simulink library "hapsrav_library"  (R2017a)
settings: Solver=VariableStepAuto  StartTime=0.0  StopTime=10.0  RelTol=1e-3
values from neighbouring files (symbols this model uses):
  absorb_h = 0:100:40000    [EnergySim.m]
  Adisk = pi * v.R_prop^2    [EnergySim.m]
  alpha_h = absorb_h    [EnergySim.m]
  aoa_data = zeros(n_cl, n)    [EnergySim.m]
  cl_bp = linspace(min_cl, max_cl,n_cl)    [EnergySim.m]
  D = [1       -.0065      288.15          0                   101325 ... (first row only)    [EnergySim.m]    (also in msn_params.m = sqrt((from_x - to_x)^2 + (from_y - to_y)^2); solar_vector.m = time.day + ut_time)
  d2r = pi / 180    (= 0.0174532925199)    [EnergySim.m]    (also in example1.m; example2.m; example3.m; example4.m)
  d_init = sqrt(dx*dx + dy*dy)    [EnergySim.m]    (also in msn_init.m)
  dchi0 = atan2(sin(dchi0), cos(dchi0))    [EnergySim.m]    (also in msn_init.m)
  dT = 0.5    [EnergySim.m]
  dT_fixed = 0.5    [EnergySim.m]
  dT_trig = 30    [EnergySim.m]
  earth_rho = 6378137.0    (= 6378137)    [EnergySim.m]
  fp = solarFP(p.orbit_rho, p.min_axis, p.orbit_dir, ic.x_ctr, ic.y_ctr, sun_az_0)    [EnergySim.m]    (also in load_fp.m = gid_tc(msn_idx).fp; solarFP.m = [1	6	2	nul eul 0	0	0	0	1	0)
  fp_coords = [x_entry y_entry]    [msn_params.m]
  fp_courses = [chi_adj nxt_chi dchi]    [msn_params.m]
  g = 9.80665    [EnergySim.m]
  Gsolar = 1367    [EnergySim.m]
  k = k+1    (= 5)    [EnergySim.m]
  K = D(:,2)    [EnergySim.m]
  lat_init = ic.lat_init_deg * obj.d2r    [EnergySim.m]
  M = time.month    [solar_vector.m]
  max_cl = max(cl_data(:))    [EnergySim.m]
  min_cl = min(cl_data(:))    [EnergySim.m]
  ND2 = load(fullfile(pwd,'nd2_data.mat'))    [EnergySim.m]    (also in nd2_data.mat = [0.0999999999999 0.200000000001 0.3 0.4 0.499999999998 0.700)
  next_init = fp(init_wp, 3)    [EnergySim.m]    (also in msn_init.m)
  pE_init = ic.pE_init    [EnergySim.m]
  pN_init = ic.pN_init    [EnergySim.m]
  r2d = 180 / pi    (= 57.2957795131)    [EnergySim.m]    (also in example1.m; example2.m; example3.m; example4.m)
  rho_SL = 1.225    [EnergySim.m]
  S = 110.4    [EnergySim.m]
  thr_lo_lim = 0.0    (= 0)    [EnergySim.m]
  time_init = struct('year', time.year, 'month', time.month,                  'day', time.day, 'hour', time.hour, 'min', time.min,                  'UTC', time.UTC)    [EnergySim.m]
  to_init = fp(init_wp, 1)    [EnergySim.m]    (also in msn_init.m)
  vgnd_init = sqrt(Vg)    [EnergySim.m]
  vtas_init = veas_init * sqrt(rho_sl/rho_alt)    [EnergySim.m]
  w_alt = 2.0 * w_alt    [EnergySim.m]
  w_xtrack = 2.0 * w_xtrack    [EnergySim.m]
undefined symbols (not defined in the file or in its folder): alpha, alpha_bp, alpha_circ, alt0_rate_init, alt_bp, alt_cmd_mode, alt_init, alt_lim_h, alt_lim_l, alt_rt_lim_periodic, cd_data, charge_eff, chi0_rate_init, chi_cmd_mode, chi_inf, chi_init, cl_data, discharge_eff, DiscIntNeverNeededParam, E_batt_max, E_init, Earth, enableFuzzyLogic, entry_init, epsln, epsln_circ, exit_init, f8_azimuth_offset, fig_eight_time, fp0, fp_coords0, fp_courses0, gamma_lim, hold_time, k_c, K_circ, lat_init_deg, lon_init_deg, max_alpha_bp, max_alt_bp, min_alpha_bp, min_alt_bp, min_axis, motor_eff, mppt_eff, num_motors, orb_dir_init, orb_len_init, orbit_dir, orbit_rho, P_acc, panel_eff, panel_vecs, phi_0, phi_lim, phi_lim_alt, phi_lim_alt_max, phi_lim_alt_min, phi_rt_lim, prop_eff_scale ... (+39)
libraries: simulink x59, hapsrav_library x9, fuzblock x3, atmospheric_library x1, aerolibtransform2 x1
(part 1 of 6)
settings Model: Creator=benthomsen  LastModifiedBy=marriott

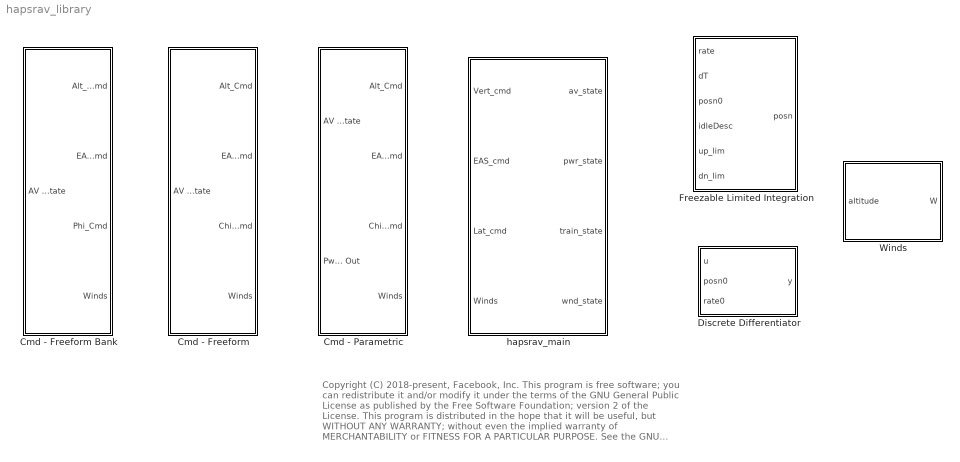
== system hapsrav_library ==
  note: Copyright (C) 2018-present, Facebook, Inc.
      |
      | This program is free software; you can redistribute it and/or modify
      | it under the terms of the GNU General Public License as published by
      | the Free Software Foundation; version 2 of the License.
      |
      | This program is distributed in the hope that it will be useful,
      | but WITHOUT ANY WARRANTY; without even the implied warranty of
      | MERCHANTABILITY or FITNESS FOR A PARTICULAR PURPOSE. See the
      | GNU General Public License for more details.
      |
      | You should have received a copy of the GNU General Public License along
      | with this program; if not, write to the Free Software Foundation, Inc.,
      | 51 Franklin Street, Fifth Floor, Boston, MA 02110-1301 USA.
  Cmd - Freeform : Subsystem
  Cmd - Freeform Bank : Subsystem
  Cmd - Parametric : Subsystem
  Discrete Differentiator : Subsystem
  Freezable Limited Integration : Subsystem
  Winds : Subsystem
  hapsrav_main : Subsystem

== system hapsrav_library/Cmd - Freeform ==
  AV State : Inport
  Alt Cmd : Subsystem
  Chi Cmd : Subsystem
  Demux1 : Demux  Outputs=28
  EAS Cmd : Subsystem
  Terminator{,1..8,10..17,19..27} (26 alike) : Terminator
  Unit Delay : UnitDelay  InitialCondition=alt_init  SampleTime=-1
  Unit Delay1 : UnitDelay  InitialCondition=chi_init  SampleTime=-1
  Winds1 : hapsrav_library/Winds
  Alt_Cmd : Outport
  EAS_Cmd : Outport  Port=2
  Chi_Cmd : Outport  Port=3
  Winds : Outport  Port=4
  wires:
  Demux1/15 -> Terminator12/1
  [alt] -> Alt Cmd/1(alt)
  Demux1/18 -> Terminator15/1
  Demux1/22 -> Terminator19/1
  Demux1/6 -> Terminator4/1
  Demux1/23 -> Terminator20/1
  Demux1/9 -> Terminator7/1
  Demux1/3 -> Terminator1/1
  Demux1/7 -> Terminator5/1
  Demux1/12 -> Unit Delay/1
  [chi] -> Chi Cmd/1(chi)
  Demux1/13 -> Terminator10/1
  Demux1/5 -> Terminator3/1
  Demux1/2 -> Terminator/1
  Demux1/20 -> Terminator17/1
  Demux1/24 -> Terminator21/1
  Demux1/10 -> Terminator8/1
  AV State/1 -> Demux1/1
  Demux1/8 -> Terminator6/1
  Demux1/16 -> Terminator13/1
  Demux1/14 -> Terminator11/1
  Demux1/19 -> Terminator16/1
  Demux1/17 -> Terminator14/1
  Demux1/4 -> Terminator2/1
  Demux1/21 -> Unit Delay1/1
  Alt Cmd/1(alt cmd) -> Alt_Cmd/1
  EAS Cmd/1(eas_cmd) -> EAS_Cmd/1
  Chi Cmd/1(chi_cmd) -> Chi_Cmd/1
  Unit Delay/1 -> [alt]
  Unit Delay1/1 -> [chi]
  Winds1/1 -> Winds/1
  [alt] -> Winds1/1
  Demux1/28 -> Terminator25/1
  Demux1/27 -> Terminator24/1
  Demux1/26 -> Terminator23/1
  Demux1/25 -> Terminator22/1
  Demux1/11 -> Terminator26/1
  Demux1/1 -> Terminator27/1

== system hapsrav_library/Cmd - Freeform Bank ==
  AV State : Inport
  Demux1 : Demux  Outputs=28
  Terminator{,1..26} (27 alike) : Terminator
  Unit Delay : UnitDelay  InitialCondition=alt_init  SampleTime=-1
  Winds1 : hapsrav_library/Winds
  alt_rt_cmd : FromWorkspace  VariableName=alt_rt_cmd  SampleTime=0
  alt_rt_cmd1 : FromWorkspace  VariableName=phi_cmd  SampleTime=0
  eas_cmd_ : FromWorkspace  VariableName=eas_cmd  SampleTime=0
  Alt_Rt_Cmd : Outport
  EAS_Cmd : Outport  Port=2
  Phi_Cmd : Outport  Port=3
  Winds : Outport  Port=4
  wires:
  alt_rt_cmd1/1 -> Phi_Cmd/1
  eas_cmd_/1 -> EAS_Cmd/1
  alt_rt_cmd/1 -> Alt_Rt_Cmd/1
  Demux1/22 -> Terminator19/1
  Demux1/7 -> Terminator5/1
  Demux1/9 -> Terminator7/1
  Demux1/21 -> Terminator18/1
  Demux1/4 -> Terminator2/1
  Demux1/14 -> Terminator11/1
  Demux1/17 -> Terminator14/1
  Demux1/19 -> Terminator16/1
  AV State/1 -> Demux1/1
  Demux1/16 -> Terminator13/1
  Demux1/8 -> Terminator6/1
  Demux1/24 -> Terminator21/1
  Demux1/10 -> Terminator8/1
  Demux1/20 -> Terminator17/1
  Demux1/13 -> Terminator10/1
  Demux1/5 -> Terminator3/1
  Demux1/15 -> Terminator12/1
  Demux1/23 -> Terminator20/1
  Demux1/2 -> Terminator/1
  Demux1/3 -> Terminator1/1
  Demux1/18 -> Terminator15/1
  Demux1/6 -> Terminator4/1
  Demux1/11 -> Terminator22/1
  Winds1/1 -> Winds/1
  Unit Delay/1 -> Winds1/1
  Demux1/1 -> Terminator9/1
  Demux1/12 -> Unit Delay/1
  Demux1/25 -> Terminator23/1
  Demux1/26 -> Terminator24/1
  Demux1/27 -> Terminator25/1
  Demux1/28 -> Terminator26/1

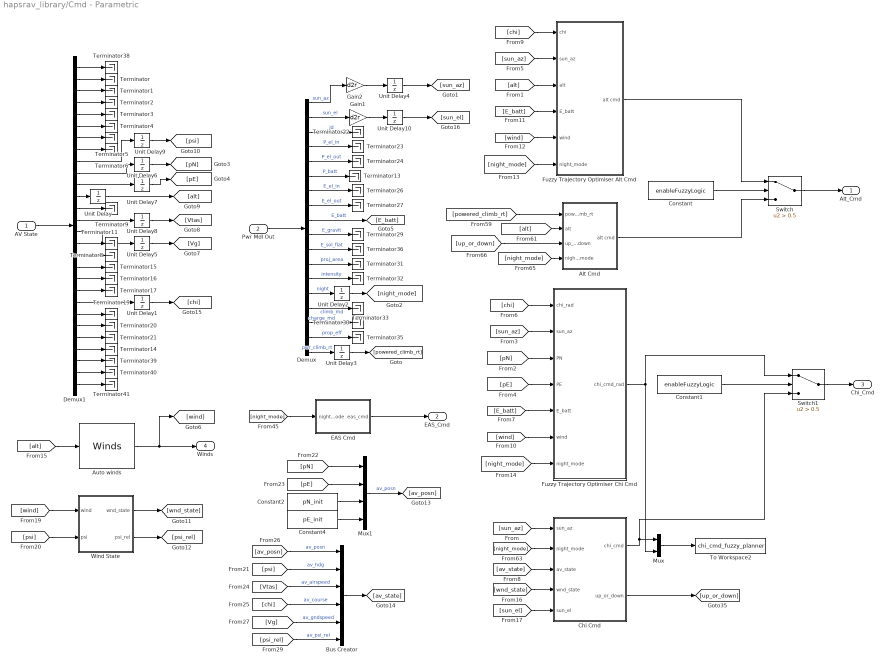
== system hapsrav_library/Cmd - Parametric ==
  AV State : Inport
  Pwr Mdl Out : Inport  Port=2
  Alt Cmd : Subsystem
  Auto winds : hapsrav_library/Winds
  Bus Creator : BusCreator  Inputs='av_posn','av_hdg','av_airspeed','av_course','av_gndspeed','av_psi_rel'
  Chi Cmd : Subsystem
  Constant : Constant  Value=enableFuzzyLogic
  Constant1 : Constant  Value=enableFuzzyLogic
  Constant2 : Constant  Value=pN_init
  Constant4 : Constant  Value=pE_init
  Demux : Demux  Outputs=18
  Demux1 : Demux  Outputs=28
  EAS Cmd : Subsystem
  Fuzzy Trajectory Optimiser Alt Cmd : Subsystem
  Fuzzy Trajectory Optimiser Chi Cmd : Subsystem
  Gain1 : Gain  Gain=d2r
  Gain2 : Gain  Gain=d2r
  Mux : Mux  Inputs=2
  Mux1 : Mux
  Switch : Switch  Criteria=u2 > Threshold  Threshold=0.5
  Switch1 : Switch  Criteria=u2 > Threshold  Threshold=0.5
  Terminator{,1..6,8..9,11,13..17,19..24,26..27,29..33,35..36,38..41} (34 alike) : Terminator
  To Workspace2 : ToWorkspace  VariableName=chi_cmd_fuzzy_planner  SampleTime=-1
  Unit Delay : UnitDelay  InitialCondition=alt_init  SampleTime=-1
  Unit Delay1 : UnitDelay  InitialCondition=chi_init  SampleTime=-1
  Unit Delay10 : UnitDelay  InitialCondition=sun_el_0  SampleTime=-1
  Unit Delay2 : UnitDelay  SampleTime=-1
  Unit Delay3 : UnitDelay  SampleTime=-1
  Unit Delay4 : UnitDelay  InitialCondition=sun_az_0  SampleTime=-1
  Unit Delay5 : UnitDelay  InitialCondition=vgnd_init  SampleTime=-1
  Unit Delay6 : UnitDelay  InitialCondition=pN_init  SampleTime=-1
  Unit Delay7 : UnitDelay  InitialCondition=pE_init  SampleTime=-1
  Unit Delay8 : UnitDelay  InitialCondition=vtas_init  SampleTime=-1
  Unit Delay9 : UnitDelay  InitialCondition=psi_0  SampleTime=-1
  Wind State : Subsystem
  Alt_Cmd : Outport
  EAS_Cmd : Outport  Port=2
  Chi_Cmd : Outport  Port=3
  Winds : Outport  Port=4
  wires:
  Gain1/1 -> Unit Delay10/1
  Demux/2 -> Gain1/1  "sun_el"
  Gain2/1 -> Unit Delay4/1
  Demux/1 -> Gain2/1  "sun_az"
  [sun_el] -> Chi Cmd/5(sun_el)
  Unit Delay10/1 -> [sun_el]
  [wnd_state] -> Chi Cmd/4(wnd_state)
  [av_state] -> Chi Cmd/3(av_state)
  [psi_rel] -> Bus Creator/6  "av_psi_rel"
  [av_posn] -> Bus Creator/1  "av_posn"
  [Vg] -> Bus Creator/5  "av_gndspeed"
  [chi] -> Bus Creator/4  "av_course"
  Bus Creator/1 -> [av_state]
  [psi] -> Bus Creator/2  "av_hdg"
  [Vtas] -> Bus Creator/3  "av_airspeed"
  [pN] -> Mux1/1
  [pE] -> Mux1/2
  Mux1/1 -> [av_posn]  "av_posn"
  Constant4/1 -> Mux1/4
  Constant2/1 -> Mux1/3
  Wind State/2(psi_rel) -> [psi_rel]
  [psi] -> Wind State/2(psi)
  Wind State/1(wnd_state) -> [wnd_state]
  [wind] -> Wind State/1(wind)
  Unit Delay9/1 -> [psi]
  Unit Delay8/1 -> [Vtas]
  Demux1/18 -> Terminator15/1
  AV State/1 -> Demux1/1
  Demux1/9 -> Unit Delay9/1
  [night_mode] -> Alt Cmd/4(night_mode)
  [up_or_down] -> Alt Cmd/3(up_or_down)
  Demux1/23 -> Terminator20/1
  [sun_az] -> Chi Cmd/1(sun_az)
  Demux1/17 -> Terminator8/1
  [night_mode] -> EAS Cmd/1(night_mode)
  Demux1/20 -> Terminator17/1
  Demux1/19 -> Terminator16/1
  Chi Cmd/2(up_or_down) -> [up_or_down]
  [powered_climb_rt] -> Alt Cmd/1(powered_climb_rt)
  Demux1/22 -> Terminator19/1
  [alt] -> Alt Cmd/2(alt)
  Demux1/4 -> Terminator2/1
  Demux1/7 -> Terminator5/1
  Demux1/5 -> Terminator3/1
  Demux1/8 -> Terminator6/1
  Demux1/10 -> Unit Delay6/1
  Demux1/2 -> Terminator/1
  Demux1/24 -> Terminator21/1
  Demux1/3 -> Terminator1/1
  Demux1/6 -> Terminator4/1
  [night_mode] -> Chi Cmd/2(night_mode)
  EAS Cmd/1(eas_cmd) -> EAS_Cmd/1
  Auto winds/1 -> [wind], Winds/1
  Unit Delay/1 -> [alt]
  Unit Delay1/1 -> [chi]
  Demux/11 -> Terminator36/1  "E_sol_flat"
  Demux/17 -> Terminator35/1  "prop_eff"
  Demux/14 -> Unit Delay2/1  "night"
  Demux/16 -> Terminator30/1  "charge_md"
  Demux/3 -> Terminator22/1  "jd"
  Pwr Mdl Out/1 -> Demux/1
  Demux/12 -> Terminator31/1  "proj_area"
  Demux/4 -> Terminator23/1  "P_el_in"
  Demux/5 -> Terminator24/1  "P_el_out"
  Demux/18 -> Unit Delay3/1  "pwr_climb_rt"
  Demux/13 -> Terminator32/1  "intensity"
  Demux/7 -> Terminator26/1  "E_el_in"
  Demux/15 -> Terminator33/1  "climb_md"
  Demux/8 -> Terminator27/1  "E_el_out"
  Demux/10 -> Terminator29/1  "E_gravit"
  Demux/9 -> [E_batt]  "E_batt"
  Demux/6 -> Terminator13/1  "P_batt"
  Unit Delay2/1 -> [night_mode]
  Unit Delay3/1 -> [powered_climb_rt]
  Unit Delay4/1 -> [sun_az]
  [chi] -> Fuzzy Trajectory Optimiser Alt Cmd/1(chi)
  [sun_az] -> Fuzzy Trajectory Optimiser Alt Cmd/2(sun_az)
  [alt] -> Fuzzy Trajectory Optimiser Alt Cmd/3(alt)
  Demux1/16 -> Terminator11/1
  Demux1/15 -> Unit Delay5/1
  Demux1/13 -> Terminator9/1
  Demux1/14 -> Unit Delay8/1
  [sun_az] -> Fuzzy Trajectory Optimiser Chi Cmd/2(sun_az)
  Mux/1 -> To Workspace2/1
  Constant/1 -> Switch/2
  Switch/1 -> Alt_Cmd/1
  Fuzzy Trajectory Optimiser Alt Cmd/1(alt cmd) -> Switch/1
  Alt Cmd/1(alt cmd) -> Switch/3
  Fuzzy Trajectory Optimiser Chi Cmd/1(chi_cmd_rad) -> Switch1/1, Mux/2
  Constant1/1 -> Switch1/2
  Switch1/1 -> Chi_Cmd/1
  Chi Cmd/1(chi_cmd) -> Switch1/3, Mux/1
  Demux1/12 -> Unit Delay/1
  Demux1/1 -> Terminator38/1
  Demux1/11 -> Unit Delay7/1
  Demux1/21 -> Unit Delay1/1
  Demux1/28 -> Terminator41/1
  Demux1/27 -> Terminator40/1
  Demux1/26 -> Terminator39/1
  Demux1/25 -> Terminator14/1
  [chi] -> Fuzzy Trajectory Optimiser Chi Cmd/1(chi_rad)
  [pN] -> Fuzzy Trajectory Optimiser Chi Cmd/3(PN)
  [pE] -> Fuzzy Trajectory Optimiser Chi Cmd/4(PE)
  [wind] -> Fuzzy Trajectory Optimiser Chi Cmd/6(wind)
  [E_batt] -> Fuzzy Trajectory Optimiser Chi Cmd/5(E_batt)
  [night_mode] -> Fuzzy Trajectory Optimiser Chi Cmd/7(night_mode)
  [E_batt] -> Fuzzy Trajectory Optimiser Alt Cmd/4(E_batt)
  [wind] -> Fuzzy Trajectory Optimiser Alt Cmd/5(wind)
  [night_mode] -> Fuzzy Trajectory Optimiser Alt Cmd/6(night_mode)
  [alt] -> Auto winds/1
  Unit Delay5/1 -> [Vg]
  Unit Delay6/1 -> [pN]
  Unit Delay7/1 -> [pE]

== system hapsrav_library/Discrete Differentiator ==
  u : Inport
  posn0 : Inport  Port=2
  rate0 : Inport  Port=3
  A : Gain  Gain=sys_lpf_A
  B : Gain  Gain=sys_lpf_B
  C : Gain  Gain=sys_lpf_C
  C1 : Gain  Gain=1/dT
  D : Gain  Gain=sys_lpf_D
  Delay : Delay  DelayLength=1  InitialConditionSource=Input port
      settings: InputPortMap=u0,p4
  Delay1 : Delay  DelayLength=1  InitialConditionSource=Input port
      settings: InputPortMap=u0,p4
  Product : Product
  Sum : Sum  Inputs=|++
  Sum1 : Sum  Inputs=|++
  Sum2 : Sum  Inputs=|+-
  x0 : Constant  Value=sys_lpf_x0
  y : Outport
  wires:
  Sum2/1 -> C1/1
  Delay1/1 -> Sum2/2
  posn0/1 -> Delay1/2
  u/1 -> Delay1/1, Sum2/1
  Delay/1 -> A/1, C/1
  Sum/1 -> Delay/1
  Sum1/1 -> y/1
  A/1 -> Sum/2
  [DuDt] -> B/1, D/1
  rate0/1 -> Product/2
  B/1 -> Sum/1
  D/1 -> Sum1/2
  x0/1 -> Product/1
  Product/1 -> Delay/2
  C/1 -> Sum1/1
  C1/1 -> [DuDt]

== system hapsrav_library/Freezable Limited Integration ==
  rate : Inport
  dT : Inport  Port=2
  posn0 : Inport  Port=3
  idleDesc : Inport  Port=4
  up_lim : Inport  Port=5
  dn_lim : Inport  Port=6
  Constant : Constant  Value=0
  Delay1 : Delay  DelayLength=1  InitialConditionSource=Input port
      settings: InputPortMap=u0,p4
  Delay2 : Delay  DelayLength=1  InitialConditionSource=Input port  InitialCondition=0
      settings: InputPortMap=u0,p4
  Delay3 : Delay  DelayLength=1  InitialConditionSource=Input port
      settings: InputPortMap=u0,p4
  Limited Integration : MATLAB Function  TreatAsAtomicUnit=on
  Switch : Switch  Threshold=1
  Switch1 : Switch  Threshold=1
  posn : Outport
  wires:
  up_lim/1 -> Limited Integration/3(uplim)
  rate/1 -> Limited Integration/1(u)
  Delay1/1 -> Limited Integration/5(x0)
  Limited Integration/2(x1) -> Delay1/1
  Limited Integration/1(y0) -> Switch/3, posn/1
  dT/1 -> Limited Integration/2(T)
  idleDesc/1 -> Delay2/1
  Delay2/1 -> [idle_desc]
  [idle_desc] -> Switch/2
  [idle_desc] -> Switch1/2
  Switch/1 -> Delay3/1
  Delay3/1 -> Switch/1, [desc_lim]
  posn0/1 -> [posn0]
  [posn0] -> Delay1/2
  [posn0] -> Delay3/2
  dn_lim/1 -> Switch1/3
  [desc_lim] -> Switch1/1
  Switch1/1 -> Limited Integration/4(lolim)
  Constant/1 -> Delay2/2

== system hapsrav_library/Winds ==
  altitude : Inport
  Constant : Constant  Value=TEST_WINDS
  Constant Winds : Subsystem
  Logical Operator : Logic  Operator=NOT  AllPortsSameDT=off  OutDataTypeStr=boolean
  Merge : Merge
  Test Winds : Subsystem
  wdir_level : Constant  Value=wdir_level
  wmag_level : Constant  Value=wmag_level
  W : Outport
  wires:
  wmag_level/1 -> Test Winds/2(wmag_level)
  wdir_level/1 -> Test Winds/3(wdir_level)
  altitude/1 -> Test Winds/1(altitude)
  Merge/1 -> W/1
  Constant Winds/1(W) -> Merge/1
  Test Winds/1(W) -> Merge/2
  Constant/1 -> Test Winds/Enable, Logical Operator/1
  Logical Operator/1 -> Constant Winds/Enable

== system hapsrav_library/hapsrav_main ==
  Vert_cmd : Inport  PortDimensions=1
  EAS_cmd : Inport  Port=2  PortDimensions=1
  Lat_cmd : Inport  Port=3  PortDimensions=1
  Winds : Inport  Port=4  PortDimensions=3
  Kinematic 6DOF : Subsystem
  Outputs : Subsystem
  av_state : Outport
  pwr_state : Outport  Port=2
  train_state : Outport  Port=3
  wnd_state : Outport  Port=4
  wires:
  Kinematic 6DOF/2(pwr_state) -> Outputs/2(Pwr State)
  Winds/1 -> Kinematic 6DOF/4(Winds)
  Lat_cmd/1 -> Kinematic 6DOF/3(Lat_cmd)
  EAS_cmd/1 -> Kinematic 6DOF/2(EAS_cmd)
  Vert_cmd/1 -> Kinematic 6DOF/1(Vert_cmd)
  Kinematic 6DOF/1(av_state) -> Outputs/1(AV State)
  Outputs/1(simOut) -> av_state/1
  Outputs/2(pwrOut) -> pwr_state/1
  Outputs/3(TrainOut) -> train_state/1
  Kinematic 6DOF/3(wnd_state) -> wnd_state/1

== system hapsrav_library/Cmd - Freeform/Alt Cmd ==
  alt : Inport
  Abs : Abs
  Compare To Constant : simulink/Logic and Bit Operations/Compare To Constant  relop=>  const=50  OutDataTypeStr=boolean
  Delay1 : Delay  DelayLength=1  InitialCondition=alt_init
  Discrete-Time Integrator : DiscreteIntegrator  IntegratorMethod=Integration: Trapezoidal  ExternalReset=rising  InitialConditionSource=external  InitialConditionSetting=State (most efficient)  SampleTime=-1  ICPrevOutput=DiscIntNeverNeededParam  ICPrevScaledInput=DiscIntNeverNeededParam
  IC : InitialCondition  Value=alt_init
  Sum : Sum  Inputs=|+-
  To Workspace : ToWorkspace  VariableName=alt_cmd  SampleTime=-1
  alt_rt_cmd : FromWorkspace  VariableName=alt_rt_cmd  SampleTime=0
  alt cmd : Outport
  wires:
  Compare To Constant/1 -> Discrete-Time Integrator/2  "trigger a reset (anti-windup)"
  Sum/1 -> Abs/1
  alt_rt_cmd/1 -> Discrete-Time Integrator/1
  alt/1 -> IC/1
  Discrete-Time Integrator/1 -> Delay1/1
  Delay1/1 -> To Workspace/1, alt cmd/1, Discrete-Time Integrator/3, Sum/2
  Abs/1 -> Compare To Constant/1
  IC/1 -> Sum/1

== system hapsrav_library/Cmd - Freeform/Chi Cmd ==
  chi : Inport
  Abs : Abs
  Compare To Constant : simulink/Logic and Bit Operations/Compare To Constant  relop=>  const=2  OutDataTypeStr=boolean
  Delay1 : Delay  DelayLength=1  InitialCondition=chi_init
  Discrete-Time Integrator : DiscreteIntegrator  IntegratorMethod=Integration: Trapezoidal  ExternalReset=rising  InitialConditionSource=external  InitialConditionSetting=State (most efficient)  SampleTime=-1  ICPrevOutput=DiscIntNeverNeededParam  ICPrevScaledInput=DiscIntNeverNeededParam
  IC : InitialCondition  Value=chi_init
  Sum : Sum  Inputs=|+-
  To Workspace : ToWorkspace  VariableName=chi_cmd  SampleTime=-1
  alt_rt_cmd : FromWorkspace  VariableName=chi_rt_cmd  SampleTime=0
  chi_cmd : Outport
  wires:
  chi/1 -> IC/1
  Delay1/1 -> To Workspace/1, chi_cmd/1, Discrete-Time Integrator/3, Sum/2
  alt_rt_cmd/1 -> Discrete-Time Integrator/1
  Abs/1 -> Compare To Constant/1
  Discrete-Time Integrator/1 -> Delay1/1
  Sum/1 -> Abs/1
  Compare To Constant/1 -> Discrete-Time Integrator/2  "trigger a reset (anti-windup)"
  IC/1 -> Sum/1

== system hapsrav_library/Cmd - Freeform/EAS Cmd ==
  eas_cmd_ : FromWorkspace  VariableName=eas_cmd  SampleTime=0
  eas_cmd : Outport
  wires:
  eas_cmd_/1 -> eas_cmd/1

== system hapsrav_library/Cmd - Parametric/Alt Cmd ==
  powered_climb_rt : Inport
  alt : Inport  Port=2
  up_or_down : Inport  Port=3
  night_mode : Inport  Port=4
  Compare To Constant : simulink/Logic and Bit Operations/Compare To Constant  relop===  const=1  OutDataTypeStr=boolean
  Compare To Constant2 : simulink/Logic and Bit Operations/Compare To Constant  relop===  const=2  OutDataTypeStr=boolean
  Constant : Constant  Value=alt_cmd_mode
  Constant2 : Constant
  Merge : Merge
  Periodic Climb/Glide : Subsystem
  Power-Limited Climb : Subsystem
  Scope : Scope
  Switch : Switch  Criteria=u2 ~= 0
  To Workspace : ToWorkspace  VariableName=alt_cmd  SampleTime=-1
  alt cmd : Outport
  wires:
  Merge/1 -> Scope/1, To Workspace/1, alt cmd/1
  powered_climb_rt/1 -> Power-Limited Climb/1(climb_rt)
  Switch/1 -> Compare To Constant2/1, Compare To Constant/1
  Compare To Constant/1 -> Power-Limited Climb/Enable
  Power-Limited Climb/1(alt_cmd) -> Merge/1
  Compare To Constant2/1 -> Periodic Climb/Glide/Enable
  Periodic Climb/Glide/1(alt_cmd) -> Merge/2
  up_or_down/1 -> Periodic Climb/Glide/1(up_or_down)
  night_mode/1 -> [night_mode]
  alt/1 -> [alt]
  [night_mode] -> Switch/2
  Constant/1 -> Switch/3
  Constant2/1 -> Switch/1
  [alt] -> Power-Limited Climb/2(alt)
  [alt] -> Periodic Climb/Glide/2(alt)

== system hapsrav_library/Cmd - Parametric/Chi Cmd ==
  sun_az : Inport
  night_mode : Inport  Port=2
  av_state : Inport  Port=3
  wnd_state : Inport  Port=4
  sun_el : Inport  Port=5
  Bus Selector : BusSelector  OutputSignals=av_hdg
  Circular Vector Fields : Subsystem  TreatAsAtomicUnit=on
  Compare To Constant1 : simulink/Logic and Bit Operations/Compare To Constant  relop===  const=4  OutDataTypeStr=boolean
  Compare To Constant2 : simulink/Logic and Bit Operations/Compare To Constant  relop===  const=5  OutDataTypeStr=boolean
  Compare To Constant3 : simulink/Logic and Bit Operations/Compare To Constant  relop===  const=3  OutDataTypeStr=boolean
  Constant2 : Constant  Value=2*pi
  Constant3 : Constant  Value=chi_cmd_mode
  Delay1 : Delay  DelayLength=1  InitialCondition=chi_init
  Flight Plan : Subsystem  TreatAsAtomicUnit=on
  Math Function1 : Math  Operator=mod  SaturateOnIntegerOverflow=on
  Merge1 : Merge  Inputs=3
  Mux4 : Mux  Inputs=2
  Scope : Scope
  Subsystem : Subsystem
  To Workspace : ToWorkspace  VariableName=chi_cmd  SampleTime=-1
  To Workspace3 : ToWorkspace  VariableName=chi_cmd_param  SampleTime=-1
  chi_cmd : Outport
  up_or_down : Outport  Port=2
  tag scope: chi_cmd=global
  wires:
  [sun_el_rad] -> Flight Plan/4(sun_el)
  sun_el/1 -> [sun_el_rad]
  Bus Selector/1 -> [chi]  "<av_hdg>"
  [av_state] -> Bus Selector/1
  [sun_az_rad] -> Flight Plan/3(sun_az)
  wnd_state/1 -> Flight Plan/2(wnd_state)
  [av_state] -> Flight Plan/1(av_state)
  Flight Plan/1(chi_ref) -> Merge1/2
  [av_state] -> Circular Vector Fields/1(av_state)
  av_state/1 -> [av_state]
  [chi_cmd_mode] -> Compare To Constant2/1
  Compare To Constant2/1 -> Flight Plan/Enable
  Compare To Constant1/1 -> Circular Vector Fields/Enable
  [chi_cmd_mode] -> Compare To Constant1/1
  Compare To Constant3/1 -> Subsystem/Enable
  [chi_cmd_mode] -> Compare To Constant3/1
  Constant3/1 -> [chi_cmd_mode]
  Subsystem/1(chi_cmd) -> Merge1/3
  Circular Vector Fields/1(chi_cmd) -> Merge1/1
  Subsystem/2(up_or_down) -> up_or_down/1
  [sun_az_rad] -> Subsystem/3(sun_az_rad)
  [chi_cmd] -> Subsystem/2(chi_cmd_in)
  [night_mode] -> Subsystem/1(night_md)
  Merge1/1 -> chi_cmd/1, Delay1/1, Scope/1, To Workspace/1, Mux4/2
  [chi] -> Mux4/1
  Mux4/1 -> Math Function1/1
  Math Function1/1 -> To Workspace3/1
  Constant2/1 -> Math Function1/2
  Delay1/1 -> [chi_cmd]
  night_mode/1 -> [night_mode]
  sun_az/1 -> [sun_az_rad]

== system hapsrav_library/Cmd - Parametric/EAS Cmd ==
  night_mode : Inport
  Constant : Constant  Value=veas_init
  Constant1 : Constant  Value=veas_night_mode
  Switch : Switch  Criteria=u2 ~= 0
  eas_cmd : Outport
  wires:
  Constant/1 -> Switch/3
  Constant1/1 -> Switch/1
  night_mode/1 -> Switch/2
  Switch/1 -> eas_cmd/1

== system hapsrav_library/Cmd - Parametric/Fuzzy Trajectory Optimiser Alt Cmd ==
  note: This is the wind vector
  chi : Inport
  sun_az : Inport  Port=2
  alt : Inport  Port=3
  E_batt : Inport  Port=4
  wind : Inport  Port=5
  night_mode : Inport  Port=6
  Alt Rate Integrator : Subsystem
  Compare To Constant1 : simulink/Logic and Bit Operations/Compare To Constant  relop=<=  const=pi  OutDataTypeStr=boolean
  Constant : Constant  Value=2*pi
  Fuzzy Logic Trajectory Planner : fuzblock/Fuzzy Logic  Controller  fis='traj_planner_altrate.fis'
  IC : InitialCondition  Value=chi_init
  "If the modulud after division is larger than pi, then sunbtract the mod results from 2*pi this procedure maps the azimuth angle difference between [0,pi]" : Switch  Criteria=u2 ~= 0
  Math Function : Math  Operator=mod  SaturateOnIntegerOverflow=on
  Mux : Mux  Inputs=2
  Subtract : Sum  Inputs=|+-
  Subtract1 : Sum  Inputs=-|+
  Terminator{,1..3} (4 alike) : Terminator
  To Workspace : ToWorkspace  VariableName=alt_cmd_fuzzy_planner  SampleTime=-1
  alt cmd : Outport
  wires:
  Fuzzy Logic Trajectory Planner/1 -> Alt Rate Integrator/1(alt_rate_cmd), Mux/1
  chi/1 -> [chi_rad], IC/1
  IC/1 -> [chi]
  [chi] -> Terminator/1
  sun_az/1 -> [sun_az_rad]
  [sun_az_rad] -> Subtract/2
  Math Function/1 -> Compare To Constant1/1, "If the modulud after division is larger than pi, then sunbtract the mod results from 2*pi this procedure maps the azimuth angle difference between [0,pi]"/1, Subtract1/1  "Azimuth difference  (rad)"
  Compare To Constant1/1 -> "If the modulud after division is larger than pi, then sunbtract the mod results from 2*pi this procedure maps the azimuth angle difference between [0,pi]"/2
  Constant/1 -> Subtract1/2, Math Function/2
  Subtract/1 -> Math Function/1
  Subtract1/1 -> "If the modulud after division is larger than pi, then sunbtract the mod results from 2*pi this procedure maps the azimuth angle difference between [0,pi]"/3
  "If the modulud after division is larger than pi, then sunbtract the mod results from 2*pi this procedure maps the azimuth angle difference between [0,pi]"/1 -> Fuzzy Logic Trajectory Planner/1
  Alt Rate Integrator/1(alt_cmd) -> Mux/2, alt cmd/1
  alt/1 -> [alt]
  [alt] -> Alt Rate Integrator/2(alt)
  Mux/1 -> To Workspace/1
  [chi_rad] -> Subtract/1
  E_batt/1 -> Terminator1/1
  wind/1 -> Terminator2/1
  night_mode/1 -> Terminator3/1

== system hapsrav_library/Cmd - Parametric/Fuzzy Trajectory Optimiser Chi Cmd ==
  note: This is the wind vector
  note: check if the aircraft is closed to the station
      |  keeping circle perimeter
  note: distance from the perimeter in meter
  chi_rad : Inport
  sun_az : Inport  Port=2
  PN : Inport  Port=3
  PE : Inport  Port=4
  E_batt : Inport  Port=5
  wind : Inport  Port=6
  night_mode : Inport  Port=7
  Abs : Abs
  Compare To Constant : simulink/Logic and Bit Operations/Compare To Constant  relop=<=  const=350  OutDataTypeStr=boolean
  Compare To Constant1 : simulink/Logic and Bit Operations/Compare To Constant  relop=<=  const=pi  OutDataTypeStr=boolean
  Constant : Constant  Value=2*pi
  Constant1 : Constant  Value=2500
  Constant2 : Constant  Value=2*pi
  Constant3 : Constant  Value=2*pi
  Discrete Derivative : simulink/Discrete/Discrete Derivative  gainval=1  ICPrevScaledInput=0.0  OutMin=[]  OutMax=[]  OutDataType=fixdt(1, 16)  OutScaling=2^-10  DoSatur=off
  Fcn : Fcn  Expr=(u(1)*u(1)+u(2)*u(2))^0.5
  Fuzzy Logic Trajectory Planner : fuzblock/Fuzzy Logic  Controller  fis='traj_planner_chi_radii.fis'
  Fuzzy Logic Trajectory Planner1 : fuzblock/Fuzzy Logic  Controller  fis='traj_planner_chi_solar.fis'
  Gain : Gain  Gain=-1
  Gain2 : Gain  Gain=1/d2r
  IC : InitialCondition  Value=chi_init
  "If the modulus after division is larger than pi, then sunbtract the mod results from 2*pi this procedure maps the azimuth angle difference between [0,pi]" : Switch  Criteria=u2 ~= 0
  "If the modulus after division is larger than pi, then sunbtract the mod results from 2*pi this procedure maps the azimuth angle difference between [0,pi]1" : Switch  Criteria=u2 > Threshold
  Math Function : Math  Operator=mod  SaturateOnIntegerOverflow=on
  Math Function1 : Math  Operator=mod  SaturateOnIntegerOverflow=on
  Math Function2 : Math  Operator=mod  SaturateOnIntegerOverflow=on
  Mux1 : Mux  Inputs=2
  Mux2 : Mux  Inputs=3
  Mux3 : Mux
  Mux4 : Mux  Inputs=2
  Subsystem : Subsystem
  Subtract : Sum  Inputs=|+-
  Subtract1 : Sum  Inputs=-|+
  Subtract2 : Sum  Inputs=-+|
  Switch : Switch  Criteria=u2 > Threshold
  Terminator{,1..3} (4 alike) : Terminator
  To Workspace1 : ToWorkspace  VariableName=chirate_cmd_vector  SampleTime=-1
  To Workspace2 : ToWorkspace  VariableName=posdiff_vector  SampleTime=-1
  To Workspace3 : ToWorkspace  VariableName=chi_cmd_fuzzy  SampleTime=-1
  chi_cmd_rad : Outport
  wires:
  sun_az/1 -> [sun_az_rad]
  Compare To Constant1/1 -> "If the modulus after division is larger than pi, then sunbtract the mod results from 2*pi this procedure maps the azimuth angle difference between [0,pi]"/2
  [sun_az_rad] -> Subtract/2
  Constant/1 -> Subtract1/2, Math Function/2
  Math Function/1 -> Compare To Constant1/1, "If the modulus after division is larger than pi, then sunbtract the mod results from 2*pi this procedure maps the azimuth angle difference between [0,pi]"/1, Subtract1/1  "Azimuth difference  (rad)"
  IC/1 -> [chi_init]
  Subtract1/1 -> "If the modulus after division is larger than pi, then sunbtract the mod results from 2*pi this procedure maps the azimuth angle difference between [0,pi]"/3
  "If the modulus after division is larger than pi, then sunbtract the mod results from 2*pi this procedure maps the azimuth angle difference between [0,pi]"/1 -> Mux2/1
  Subtract2/1 -> Mux2/2, Discrete Derivative/1, Abs/1
  PN/1 -> Mux1/1
  PE/1 -> Mux1/2
  Mux1/1 -> Fcn/1
  Fcn/1 -> Subtract2/1
  Constant1/1 -> Subtract2/2
  Mux2/1 -> Fuzzy Logic Trajectory Planner/1, Fuzzy Logic Trajectory Planner1/1
  Subsystem/1(chi_cmd_rad) -> chi_cmd_rad/1, Mux4/2
  Discrete Derivative/1 -> Mux2/3, To Workspace2/1
  chi_rad/1 -> [chi_rad], IC/1
  [chi_init] -> Terminator/1
  [chi_rad] -> Subsystem/2(chi)
  Abs/1 -> Compare To Constant/1
  Compare To Constant/1 -> Switch/2
  Switch/1 -> Mux3/3, Subsystem/1(chi_rate_cmd_rps)
  Mux3/1 -> To Workspace1/1
  Constant2/1 -> Math Function1/2
  Mux4/1 -> Math Function1/1
  [chi_rad] -> Mux4/1
  Math Function1/1 -> To Workspace3/1
  [chi_rad] -> Math Function2/1
  Constant3/1 -> Math Function2/2
  Math Function2/1 -> Subtract/1
  Fuzzy Logic Trajectory Planner/1 -> Switch/1
  Gain/1 -> "If the modulus after division is larger than pi, then sunbtract the mod results from 2*pi this procedure maps the azimuth angle difference between [0,pi]1"/1
  "If the modulus after division is larger than pi, then sunbtract the mod results from 2*pi this procedure maps the azimuth angle difference between [0,pi]1"/1 -> Mux3/1
  Subtract/1 -> "If the modulus after division is larger than pi, then sunbtract the mod results from 2*pi this procedure maps the azimuth angle difference between [0,pi]1"/2, Gain2/1, Math Function/1
  Gain2/1 -> Mux3/4
  Fuzzy Logic Trajectory Planner1/1 -> "If the modulus after division is larger than pi, then sunbtract the mod results from 2*pi this procedure maps the azimuth angle difference between [0,pi]1"/3, Mux3/2, Switch/3, Gain/1
  E_batt/1 -> Terminator1/1
  wind/1 -> Terminator2/1
  night_mode/1 -> Terminator3/1

== system hapsrav_library/Cmd - Parametric/Wind State ==
  wind : Inport
  psi : Inport  Port=2
  Demux2 : Demux  Outputs=3
  Mux1 : Mux  Inputs=2
  Product : Product
  Product1 : Product
  Rel Hdg : Subsystem
  Sqrt : Sqrt  SaturateOnIntegerOverflow=on
  Sum : Sum  Inputs=|++
  Terminator7 : Terminator
  Trigonometric Function : Trigonometry  Operator=atan2
  wnd_state : Outport
  psi_rel : Outport  Port=2
  wires:
  [Wn] -> Trigonometric Function/2
  [We] -> Trigonometric Function/1
  [Wdir] -> Rel Hdg/1(wnd_dir)
  Rel Hdg/1(rel_wnd) -> psi_rel/1
  psi/1 -> Rel Hdg/2(psi)
  [Wn] -> Product/1
  [We] -> Product1/2
  wind/1 -> Demux2/1
  Mux1/1 -> wnd_state/1
  Trigonometric Function/1 -> [Wdir]
  Demux2/3 -> Terminator7/1
  Product/1 -> Sum/1
  Sqrt/1 -> [Wspd]
  [Wdir] -> Mux1/2
  Sum/1 -> Sqrt/1
  [We] -> Product1/1
  [Wspd] -> Mux1/1
  Demux2/1 -> [Wn]
  Product1/1 -> Sum/2
  [Wn] -> Product/2
  Demux2/2 -> [We]

== system hapsrav_library/Winds/Constant Winds ==
  Enable : EnablePort
  Down : Constant  Value=Wd
  East : Constant  Value=We
  Mux : Mux  Inputs=3
  North : Constant  Value=Wn
  W : Outport
  wires:
  Down/1 -> Mux/3
  Mux/1 -> W/1
  North/1 -> Mux/1
  East/1 -> Mux/2

== system hapsrav_library/Winds/Test Winds ==
  altitude : Inport
  wmag_level : Inport  Port=2
  wdir_level : Inport  Port=3
  Enable : EnablePort
  Day : Constant  Value=wind_day
  Down : Constant  Value=Wd
  If : If  IfExpression=u1 <= 0.01
  Merge : Merge
  Merge1 : Merge
  Mux : Mux  Inputs=3
  Turn winds off at runtime : Subsystem  TreatAsAtomicUnit=on
  Winds : Subsystem  TreatAsAtomicUnit=on
  W : Outport
  wires:
  Mux/1 -> W/1
  Down/1 -> Mux/3
  [winds_on] -> Winds/Action
  Day/1 -> Winds/1(day)
  wmag_level/1 -> [wmag_level]
  [winds_off] -> Turn winds off at runtime/Action
  If/1 -> [winds_off]
  If/2 -> [winds_on]
  [wmag_level] -> If/1
  altitude/1 -> Winds/4(altitude)
  [wn_0] -> Merge/1
  [wn_1] -> Merge/2
  [we_0] -> Merge1/1
  [we_1] -> Merge1/2
  Turn winds off at runtime/1(Wn) -> [wn_0]
  Turn winds off at runtime/2(We) -> [we_0]
  Winds/1(Wn) -> [wn_1]
  Winds/2(We) -> [we_1]
  Merge1/1 -> Mux/2
  Merge/1 -> Mux/1
  [wmag_level] -> Winds/2(wmag_level)
  wdir_level/1 -> Winds/3(wdir_level)

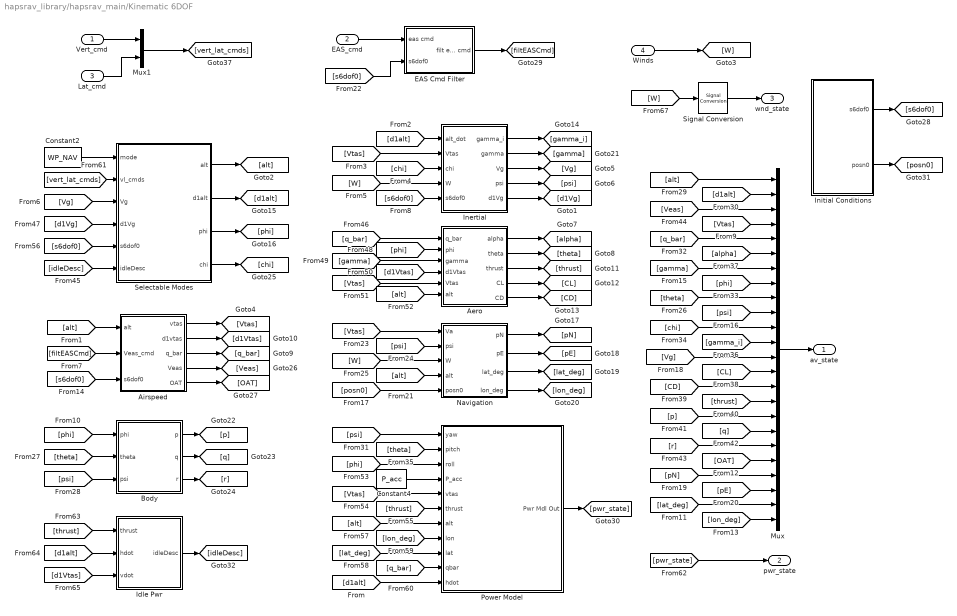
== system hapsrav_library/hapsrav_main/Kinematic 6DOF ==
  Vert_cmd : Inport
  EAS_cmd : Inport  Port=2
  Lat_cmd : Inport  Port=3
  Winds : Inport  Port=4
  Aero : Subsystem
  Airspeed : Subsystem
  Body : Subsystem
  Constant2 : Constant  Value=WP_NAV
  Constant4 : Constant  Value=P_acc
  EAS Cmd Filter : Subsystem
  Idle Pwr : Subsystem
  Inertial : Subsystem
  Initial Conditions : Subsystem
  Mux : Mux  Inputs=24
  Mux1 : Mux  Inputs=2
  Navigation : Subsystem
  Power Model : Subsystem
  Selectable Modes : Subsystem
  Signal Conversion : SignalConversion  OverrideOpt=off
  av_state : Outport
  pwr_state : Outport  Port=2
  wnd_state : Outport  Port=3
  wires:
  [s6dof0] -> Airspeed/3(s6dof0)
  [alt] -> Airspeed/1(alt)
  [filtEASCmd] -> Airspeed/2(Veas_cmd)
  Airspeed/5(OAT) -> [OAT]
  Airspeed/4(Veas) -> [Veas]
  Airspeed/3(q_bar) -> [q_bar]
  Airspeed/2(d1vtas) -> [d1Vtas]
  Airspeed/1(vtas) -> [Vtas]
  Idle Pwr/1(idleDesc) -> [idleDesc]
  [d1Vtas] -> Idle Pwr/3(vdot)
  [d1alt] -> Idle Pwr/2(hdot)
  [thrust] -> Idle Pwr/1(thrust)
  [idleDesc] -> Selectable Modes/6(idleDesc)
  Body/1(p) -> [p]
  [d1alt] -> Inertial/1(alt_dot)
  [Vtas] -> Inertial/2(Vtas)
  [chi] -> Inertial/3(chi)
  [Vtas] -> Navigation/1(Va)
  Navigation/2(pE) -> [pE]
  [phi] -> Body/1(phi)
  [theta] -> Body/2(theta)
  [psi] -> Body/3(psi)
  [W] -> Navigation/3(W)
  Inertial/1(gamma_i) -> [gamma_i]
  Inertial/4(psi) -> [psi]
  Inertial/2(gamma) -> [gamma]
  [W] -> Inertial/4(W)
  Navigation/1(pN) -> [pN]
  [psi] -> Navigation/2(psi)
  Inertial/3(Vg) -> [Vg]
  Body/2(q) -> [q]
  Body/3(r) -> [r]
  Winds/1 -> [W]
  [d1alt] -> Mux/2
  [Veas] -> Mux/3
  [Vtas] -> Mux/4
  [q_bar] -> Mux/5
  [alpha] -> Mux/6
  [gamma] -> Mux/7
  [phi] -> Mux/8
  [theta] -> Mux/9
  [psi] -> Mux/10
  [chi] -> Mux/11
  [gamma_i] -> Mux/12
  [Vg] -> Mux/13
  [CL] -> Mux/14
  [p] -> Mux/17
  [q] -> Mux/18
  [r] -> Mux/19
  Mux/1 -> av_state/1
  [alt] -> Mux/1
  [CD] -> Mux/15
  [thrust] -> Mux/16
  EAS_cmd/1 -> EAS Cmd Filter/1(eas cmd)
  EAS Cmd Filter/1(filt eas cmd) -> [filtEASCmd]
  [q_bar] -> Aero/1(q_bar)
  [phi] -> Aero/2(phi)
  [gamma] -> Aero/3(gamma)
  [d1Vtas] -> Aero/4(d1Vtas)
  [Vtas] -> Aero/5(Vtas)
  [alt] -> Aero/6(alt)
  Aero/1(alpha) -> [alpha]
  Aero/2(theta) -> [theta]
  Aero/3(thrust) -> [thrust]
  Aero/4(CL) -> [CL]
  Aero/5(CD) -> [CD]
  [alt] -> Navigation/4(alt)
  Navigation/3(lat_deg) -> [lat_deg]
  Navigation/4(lon_deg) -> [lon_deg]
  [lon_deg] -> Mux/24
  [lat_deg] -> Mux/23
  [OAT] -> Mux/20
  [pN] -> Mux/21
  [pE] -> Mux/22
  [posn0] -> Navigation/5(posn0)
  Initial Conditions/2(posn0) -> [posn0]
  Vert_cmd/1 -> Mux1/1
  Lat_cmd/1 -> Mux1/2
  Mux1/1 -> [vert_lat_cmds]
  Inertial/5(d1Vg) -> [d1Vg]
  Constant2/1 -> Selectable Modes/1(mode)
  [vert_lat_cmds] -> Selectable Modes/2(vl_cmds)
  [Vg] -> Selectable Modes/3(Vg)
  [d1Vg] -> Selectable Modes/4(d1Vg)
  [s6dof0] -> Selectable Modes/5(s6dof0)
  Selectable Modes/1(alt) -> [alt]
  Selectable Modes/2(d1alt) -> [d1alt]
  Selectable Modes/3(phi) -> [phi]
  Selectable Modes/4(chi) -> [chi]
  Initial Conditions/1(s6dof0) -> [s6dof0]
  [s6dof0] -> Inertial/5(s6dof0)
  [s6dof0] -> EAS Cmd Filter/2(s6dof0)
  [psi] -> Power Model/1(yaw)
  [d1alt] -> Power Model/11(hdot)
  [q_bar] -> Power Model/10(qbar)
  [lat_deg] -> Power Model/9(lat)
  [lon_deg] -> Power Model/8(lon)
  [alt] -> Power Model/7(alt)
  [thrust] -> Power Model/6(thrust)
  [Vtas] -> Power Model/5(vtas)
  Constant4/1 -> Power Model/4(P_acc)
  [phi] -> Power Model/3(roll)
  [theta] -> Power Model/2(pitch)
  [pwr_state] -> pwr_state/1
  [W] -> Signal Conversion/1
  Signal Conversion/1 -> wnd_state/1
  Power Model/1(Pwr Mdl Out) -> [pwr_state]

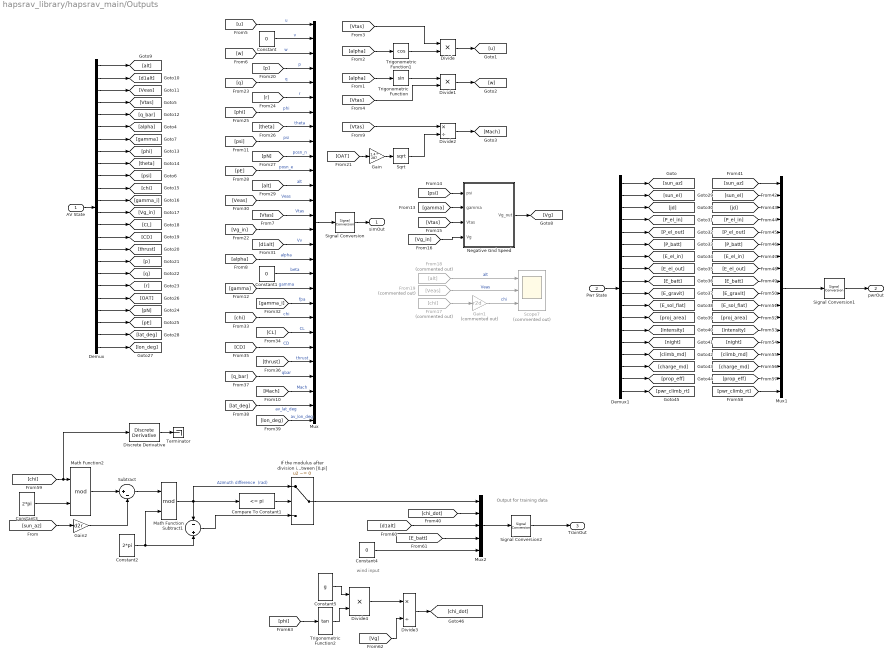
== system hapsrav_library/hapsrav_main/Outputs ==
  note: wind input
  note: Output for training data
  AV State : Inport
  Pwr State : Inport  Port=2
  Compare To Constant1 : simulink/Logic and Bit Operations/Compare To Constant  relop=<=  const=pi  OutDataTypeStr=boolean
  Constant : Constant  Value=0
  Constant1 : Constant  Value=0
  Constant2 : Constant  Value=2*pi
  Constant3 : Constant  Value=2*pi
  Constant4 : Constant  Value=0
  Constant5 : Constant  Value=g
  Demux : Demux  Outputs=24
  Demux1 : Demux  Outputs=18
  Discrete Derivative : simulink/Discrete/Discrete Derivative  gainval=1  ICPrevScaledInput=0.0  OutMin=[]  OutMax=[]  OutDataType=fixdt(1, 16)  OutScaling=2^-10  DoSatur=off
  Divide : Product  Inputs=**
  Divide1 : Product  Inputs=**
  Divide2 : Product  Inputs=*/
  Divide3 : Product  Inputs=*/
  Divide4 : Product  Inputs=**
  From17 : From  Commented=on  GotoTag=chi
  From18 : From  Commented=on  GotoTag=alt
  From19 : From  Commented=on  GotoTag=Veas
  Gain : Gain  Gain=1.4 * 287
  Gain1 : Gain  Commented=on  Gain=r2d
  Gain2 : Gain  Gain=d2r
  "If the modulus after division is larger than pi, then sunbtract the mod results from 2*pi this procedure maps the azimuth angle difference between [0,pi]" : Switch  Criteria=u2 ~= 0
  Math Function : Math  Operator=mod  SaturateOnIntegerOverflow=on
  Math Function2 : Math  Operator=mod  SaturateOnIntegerOverflow=on
  Mux : Mux  Inputs=28
  Mux1 : Mux  Inputs=18
  Mux2 : Mux  Inputs=5
  Negative Gnd Speed : Subsystem
  Scope7 : Scope  Commented=on  NumInputPorts=3
  Signal Conversion : SignalConversion  OverrideOpt=off
  Signal Conversion1 : SignalConversion  OverrideOpt=off
  Signal Conversion2 : SignalConversion  OverrideOpt=off
  Sqrt : Sqrt  SaturateOnIntegerOverflow=on
  Subtract : Sum  Inputs=|+-
  Subtract1 : Sum  Inputs=-|+
  Terminator : Terminator
  Trigonometric Function : Trigonometry
  Trigonometric Function1 : Trigonometry  Operator=cos
  Trigonometric Function2 : Trigonometry  Operator=tan
  simOut : Outport
  pwrOut : Outport  Port=2
  TrainOut : Outport  Port=3
  wires:
  [alpha] -> Trigonometric Function/1
  [alpha] -> Trigonometric Function1/1
  Trigonometric Function1/1 -> Divide/2
  [Vtas] -> Divide/1
  Trigonometric Function/1 -> Divide1/1
  [Vtas] -> Divide1/2
  Divide/1 -> [u]
  Divide1/1 -> [w]
  [u] -> Mux/1  "u"
  [w] -> Mux/3  "w"
  Constant/1 -> Mux/2  "v"
  [p] -> Mux/4  "p"
  [q] -> Mux/5  "q"
  [r] -> Mux/6  "r"
  [phi] -> Mux/7  "phi"
  [theta] -> Mux/8  "theta"
  [pN] -> Mux/10  "posn_n"
  [pE] -> Mux/11  "posn_e"
  [alt] -> Mux/12  "alt"
  [Veas] -> Mux/13  "Veas"
  [Vtas] -> Mux/14  "Vtas"
  [d1alt] -> Mux/16  "Vv"
  [alpha] -> Mux/17  "alpha"
  Constant1/1 -> Mux/18  "beta"
  [gamma_i] -> Mux/20  "fpa"
  [chi] -> Mux/21  "chi"
  [CL] -> Mux/22  "CL"
  [CD] -> Mux/23  "CD"
  [thrust] -> Mux/24  "thrust"
  [q_bar] -> Mux/25  "qbar"
  [OAT] -> Gain/1
  Gain/1 -> Sqrt/1
  [Vtas] -> Divide2/1
  Sqrt/1 -> Divide2/2
  Divide2/1 -> [Mach]
  [Mach] -> Mux/26  "Mach"
  [psi] -> Mux/9  "psi"
  [gamma] -> Mux/19  "gamma"
  [psi] -> Negative Gnd Speed/1(psi)
  [gamma] -> Negative Gnd Speed/2(gamma)
  [Vtas] -> Negative Gnd Speed/3(Vtas)
  Negative Gnd Speed/1(Vg_out) -> [Vg]
  From17/1 -> Gain1/1
  From18/1 -> Scope7/1  "alt"
  From19/1 -> Scope7/2  "Veas"
  Gain1/1 -> Scope7/3  "chi"
  AV State/1 -> Demux/1
  Demux/4 -> [Vtas]
  Demux/6 -> [alpha]
  Demux/7 -> [gamma]
  Demux/10 -> [psi]
  Demux/2 -> [d1alt]
  Demux/3 -> [Veas]
  Demux/5 -> [q_bar]
  Demux/8 -> [phi]
  Demux/9 -> [theta]
  Demux/15 -> [CD]
  Demux/16 -> [thrust]
  Demux/11 -> [chi]
  Demux/12 -> [gamma_i]
  Demux/13 -> [Vg_in]
  Demux/14 -> [CL]
  Demux/17 -> [p]
  Demux/18 -> [q]
  Demux/19 -> [r]
  Demux/20 -> [OAT]
  Demux/21 -> [pN]
  Demux/22 -> [pE]
  Demux/23 -> [lat_deg]
  Demux/24 -> [lon_deg]
  [lat_deg] -> Mux/27  "av_lat_deg"
  [lon_deg] -> Mux/28  "av_lon_deg"
  Demux/1 -> [alt]
  Mux/1 -> Signal Conversion/1
  Signal Conversion/1 -> simOut/1
  Signal Conversion1/1 -> pwrOut/1
  Gain2/1 -> Subtract/2
  Constant3/1 -> Math Function2/2
  Math Function/1 -> Compare To Constant1/1, "If the modulus after division is larger than pi, then sunbtract the mod results from 2*pi this procedure maps the azimuth angle difference between [0,pi]"/1, Subtract1/1  "Azimuth difference  (rad)"
  [chi] -> Discrete Derivative/1, Math Function2/1
  Math Function2/1 -> Subtract/1
  Subtract/1 -> Math Function/1
  Subtract1/1 -> "If the modulus after division is larger than pi, then sunbtract the mod results from 2*pi this procedure maps the azimuth angle difference between [0,pi]"/3
  Constant2/1 -> Subtract1/2, Math Function/2
  Compare To Constant1/1 -> "If the modulus after division is larger than pi, then sunbtract the mod results from 2*pi this procedure maps the azimuth angle difference between [0,pi]"/2
  Demux1/1 -> [sun_az]
  Pwr State/1 -> Demux1/1
  Demux1/2 -> [sun_el]
  Demux1/3 -> [jd]
  Demux1/4 -> [P_el_in]
  Demux1/5 -> [P_el_out]
  Demux1/6 -> [P_batt]
  Demux1/7 -> [E_el_in]
  Demux1/8 -> [E_el_out]
  Demux1/9 -> [E_batt]
  Demux1/10 -> [E_gravit]
  Demux1/11 -> [E_sol_flat]
  Demux1/12 -> [proj_area]
  Demux1/13 -> [intensity]
  Demux1/14 -> [night]
  Demux1/15 -> [climb_md]
  Demux1/16 -> [charge_md]
  Demux1/17 -> [prop_eff]
  Demux1/18 -> [pwr_climb_rt]
  [jd] -> Mux1/3
  [climb_md] -> Mux1/15
  [intensity] -> Mux1/13
  [P_el_out] -> Mux1/5
  [E_batt] -> Mux1/9
  [P_el_in] -> Mux1/4
  [proj_area] -> Mux1/12
  [sun_az] -> Mux1/1
  [P_batt] -> Mux1/6
  [E_sol_flat] -> Mux1/11
  [night] -> Mux1/14
  [E_gravit] -> Mux1/10
  [pwr_climb_rt] -> Mux1/18
  [E_el_in] -> Mux1/7
  [prop_eff] -> Mux1/17
  [sun_el] -> Mux1/2
  [E_el_out] -> Mux1/8
  [charge_md] -> Mux1/16
  Mux1/1 -> Signal Conversion1/1
  "If the modulus after division is larger than pi, then sunbtract the mod results from 2*pi this procedure maps the azimuth angle difference between [0,pi]"/1 -> Mux2/1
  [sun_az] -> Gain2/1
  Mux2/1 -> Signal Conversion2/1
  Signal Conversion2/1 -> TrainOut/1
  [chi_dot] -> Mux2/2
  [d1alt] -> Mux2/3
  [E_batt] -> Mux2/4
  Constant4/1 -> Mux2/5
  Trigonometric Function2/1 -> Divide4/2
  [phi] -> Trigonometric Function2/1
  Discrete Derivative/1 -> Terminator/1
  Constant5/1 -> Divide4/1
  Divide4/1 -> Divide3/1
  [Vg] -> Divide3/2
  Divide3/1 -> [chi_dot]
  [Vg_in] -> Mux/15
  [Vg_in] -> Negative Gnd Speed/4(Vg)

== system hapsrav_library/Cmd - Parametric/Alt Cmd/Periodic Climb//Glide ==
  up_or_down : Inport
  alt : Inport  Port=2
  Enable : EnablePort
  Abs : Abs
  Compare To Constant : simulink/Logic and Bit Operations/Compare To Constant  relop=>  const=50  OutDataTypeStr=boolean
  Delay1 : Delay  DelayLength=1  InitialCondition=alt_init
  Discrete-Time Integrator : DiscreteIntegrator  IntegratorMethod=Integration: Trapezoidal  ExternalReset=rising  InitialConditionSource=external  InitialConditionSetting=State (most efficient)  SampleTime=-1  ICPrevOutput=DiscIntNeverNeededParam  ICPrevScaledInput=DiscIntNeverNeededParam
  Gain : Gain  Gain=alt_rt_lim_periodic
  Sum : Sum  Inputs=|+-
  alt_cmd : Outport
  wires:
  Delay1/1 -> alt_cmd/1, Discrete-Time Integrator/3, Sum/2
  Compare To Constant/1 -> Discrete-Time Integrator/2  "trigger a reset (anti-windup)"
  Sum/1 -> Abs/1
  up_or_down/1 -> Gain/1
  alt/1 -> Sum/1
  Discrete-Time Integrator/1 -> Delay1/1
  Abs/1 -> Compare To Constant/1
  Gain/1 -> Discrete-Time Integrator/1

== system hapsrav_library/Cmd - Parametric/Alt Cmd/Power-Limited Climb ==
  climb_rt : Inport
  alt : Inport  Port=2
  Enable : EnablePort
  Abs : Abs
  Compare To Constant : simulink/Logic and Bit Operations/Compare To Constant  relop=>  const=50  OutDataTypeStr=boolean
  Delay1 : Delay  DelayLength=1  InitialCondition=alt_init
  Discrete-Time Integrator : DiscreteIntegrator  IntegratorMethod=Integration: Trapezoidal  ExternalReset=rising  InitialConditionSource=external  InitialConditionSetting=State (most efficient)  SampleTime=-1  ICPrevOutput=DiscIntNeverNeededParam  ICPrevScaledInput=DiscIntNeverNeededParam
  Sum : Sum  Inputs=|+-
  alt_cmd : Outport
  wires:
  Delay1/1 -> alt_cmd/1, Discrete-Time Integrator/3, Sum/2
  Compare To Constant/1 -> Discrete-Time Integrator/2  "trigger a reset (anti-windup)"
  Sum/1 -> Abs/1
  alt/1 -> Sum/1
  Discrete-Time Integrator/1 -> Delay1/1
  Abs/1 -> Compare To Constant/1
  climb_rt/1 -> Discrete-Time Integrator/1

== system hapsrav_library/Cmd - Parametric/Chi Cmd/Circular Vector Fields ==
  av_state : Inport
  Enable : EnablePort  StatesWhenEnabling=reset
  Bus Selector : BusSelector  OutputSignals=av_posn,av_course,av_gndspeed
  Constant1 : Constant  Value=x_ctr
  Constant12 : Constant  Value=k_c
  Constant2 : Constant  Value=epsln_circ
  Constant3 : Constant  Value=y_ctr
  Constant4 : Constant  Value=alpha_circ
  Constant5 : Constant  Value=K_circ
  Constant6 : Constant  Value=orbit_dir
  Constant7 : Constant  Value=orbit_rho
  Demux : Demux
  MATLAB Function1 : MATLAB Function  TreatAsAtomicUnit=on
  MATLAB Function3 : MATLAB Function  TreatAsAtomicUnit=on
  Terminator : Terminator
  Terminator1 : Terminator
  chi_cmd : Outport
  wires:
  Demux/4 -> Terminator1/1
  Demux/3 -> Terminator/1
  Demux/2 -> [av_y]
  Demux/1 -> [av_x]
  Bus Selector/1 -> Demux/1  "<av_posn>"
  Bus Selector/3 -> [Vg]  "<av_gndspeed>"
  Bus Selector/2 -> [chi]  "<av_course>"
  av_state/1 -> Bus Selector/1
  [orbit_rho] -> MATLAB Function1/6(r_c)
  Constant4/1 -> MATLAB Function3/7(alpha)
  [Vg] -> MATLAB Function3/6(Vg)
  [av_x] -> MATLAB Function1/1(av_x)
  MATLAB Function1/3(beta) -> [beta]
  [beta] -> MATLAB Function3/5(beta)
  MATLAB Function1/4(chi_d) -> [chi_d]
  [y_ctr] -> MATLAB Function1/4(y_c)
  MATLAB Function3/1(chi_cmd) -> chi_cmd/1
  Constant2/1 -> MATLAB Function3/8(e)
  MATLAB Function1/2(g) -> [rel_ang]
  Constant5/1 -> MATLAB Function3/9(K)
  Constant12/1 -> MATLAB Function1/7(k_c)
  [x_ctr] -> MATLAB Function1/3(x_c)
  [orbit_dir] -> MATLAB Function1/5(orbit_dir)
  [chi] -> MATLAB Function3/1(chi)
  [dist] -> MATLAB Function3/2(d)
  MATLAB Function1/1(d) -> [dist]
  [av_y] -> MATLAB Function1/2(av_y)
  [rel_ang] -> MATLAB Function3/3(g)
  [chi_d] -> MATLAB Function3/4(chi_d)
  Constant1/1 -> [x_ctr]
  Constant3/1 -> [y_ctr]
  Constant6/1 -> [orbit_dir]
  Constant7/1 -> [orbit_rho]

== system hapsrav_library/Cmd - Parametric/Chi Cmd/Flight Plan ==
  av_state : Inport
  wnd_state : Inport  Port=2
  sun_az : Inport  Port=3
  sun_el : Inport  Port=4
  Enable : EnablePort  StatesWhenEnabling=reset
  D2N : Subsystem
  Manual Switch : ManualSwitch  CurrentSetting=0
  Mission Command : Subsystem
  Mission Director : Subsystem
  Terminator1 : Terminator
  chi_ref : Outport
  wires:
  sun_az/1 -> Mission Director/4(sol_az)
  sun_el/1 -> Terminator1/1
  [chi_cmd] -> Manual Switch/2
  Mission Director/1(leg_state) -> [leg_state]
  [av_state] -> Mission Command/3(av_state)
  [av_state] -> D2N/2(av_state)
  Mission Director/3(nav_mode) -> [nav_mode]
  [wnd_state] -> Mission Director/3(wind_state)
  [orbit_state] -> Mission Command/1(orbit_state)
  [nav_mode] -> Mission Command/4(nav_mode)
  [chi_d] -> Manual Switch/1
  [av_state] -> Mission Director/2(av_state)
  Mission Command/1(chi_cmd) -> [chi_cmd]
  wnd_state/1 -> [wnd_state]
  [leg_state] -> Mission Command/2(leg_state)
  Mission Director/2(orbit_state) -> [orbit_state]
  av_state/1 -> [av_state]
  Manual Switch/1 -> chi_ref/1
  Mission Command/2(chi_d) -> [chi_d]
  D2N/1(av_d2n) -> Mission Director/1(d2n)
  Mission Command/3(sweep) -> Mission Director/5(sweep)
  [leg_state] -> D2N/1(leg_state)
